simulink model "ESE4481_hw2 - Copy"  (R2021a)
settings: Solver=VariableStepAuto  StartTime=0.0  StopTime=10.0  RelTol=1e-3
undefined symbols (not defined in the file or in its folder): g, J, m, omega_0, p_ned_0, Theta_0, V_b_0
libraries: vrlib x4
settings Model: Creator=tomwh  LastModifiedBy=tomwh
settings DataIOCC: ExternalInput=F_b,omega_bE,M_b

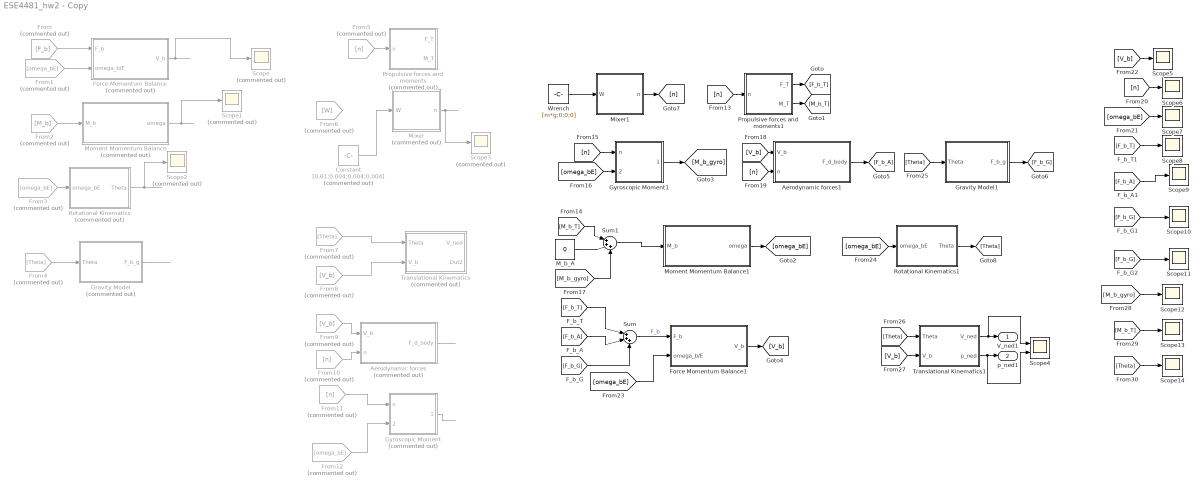
== system ESE4481_hw2 - Copy ==
  Aerodynamic forces : Subsystem  Commented=on
  Aerodynamic forces1 : Subsystem
  Constant : Constant  Commented=on  Value=[0.01;0.004;0.004;0.004]
  Force Momentum Balance : Subsystem  Commented=on
  Force Momentum Balance1 : Subsystem
  From : From  Commented=on  GotoTag=F_b
  From1 : From  Commented=on  GotoTag=omega_bE
  From10 : From  Commented=on  GotoTag=n
  From11 : From  Commented=on  GotoTag=n
  From12 : From  Commented=on  GotoTag=omega_bE
  From2 : From  Commented=on  GotoTag=M_b
  From3 : From  Commented=on  GotoTag=omega_bE
  From4 : From  Commented=on  GotoTag=Theta
  From5 : From  Commented=on  GotoTag=n
  From6 : From  Commented=on  GotoTag=W
  From7 : From  Commented=on  GotoTag=Theta
  From8 : From  Commented=on  GotoTag=V_b
  From9 : From  Commented=on  GotoTag=V_b
  Gravity Model : Subsystem  Commented=on
  Gravity Model1 : Subsystem
  Gyroscopic Moment : Subsystem  Commented=on
  Gyroscopic Moment1 : Subsystem
  M_b_A : Constant  Value=0
  Mixer : Subsystem  Commented=on
  Mixer1 : Subsystem
  Moment Momentum Balance : Subsystem  Commented=on
  Moment Momentum Balance1 : Subsystem
  Propulsive forces and moments : Subsystem  Commented=on
  Propulsive forces and moments1 : Subsystem
  Rotational Kinematics : Subsystem  Commented=on
  Rotational Kinematics1 : Subsystem
  Scope{,1..3} (4 alike) : Scope  Commented=on
  Scope{5..14} (10 alike) : Scope
  Scope4 : Scope  NumInputPorts=2
  Sum : Sum  Inputs=|+++
  Sum1 : Sum  Inputs=|+++
  Translational Kinematics : Subsystem  Commented=on
  Translational Kinematics1 : Subsystem
  Wrench : Constant  Value=[m*g;0;0;0]
  V_ned1 : Outport
  p_ned1 : Outport  Port=2
  wires:
  Force Momentum Balance/1(V_b) -> Scope/1
  From2/1 -> Moment Momentum Balance/1(M_b)
  Moment Momentum Balance/1(omega) -> Scope1/1
  Rotational Kinematics/1(Theta) -> Scope2/1
  From1/1 -> Force Momentum Balance/2(omega_b/E)
  From/1 -> Force Momentum Balance/1(F_b)
  From3/1 -> Rotational Kinematics/1(omega_bE)
  From4/1 -> Gravity Model/1(Theta)
  Gravity Model/1(F_b_g) -> ?
  From5/1 -> Propulsive forces and moments/1(n)
  Mixer/1(n) -> Scope3/1
  Constant/1 -> Mixer/1(W)
  From7/1 -> Translational Kinematics/1(Theta)
  From8/1 -> Translational Kinematics/2(V_b)
  From9/1 -> Aerodynamic forces/1(V_b)
  From10/1 -> Aerodynamic forces/2(n)
  Aerodynamic forces/1(F_d_body) -> ?
  Wrench/1 -> Mixer1/1(W)
  Mixer1/1(n) -> [n]
  [n] -> Propulsive forces and moments1/1(n)
  Propulsive forces and moments1/1(F_T) -> [F_b_T]
  Propulsive forces and moments1/2(M_T) -> [M_b_T]
  [M_b_T] -> Sum1/1
  M_b_A/1 -> Sum1/2
  From11/1 -> Gyroscopic Moment/1(n)
  From12/1 -> Gyroscopic Moment/2(omega_bE)
  Gyroscopic Moment/1(M_gyro) -> ?
  [n] -> Gyroscopic Moment1/1(n)
  Moment Momentum Balance1/1(omega) -> [omega_bE]
  [omega_bE] -> Gyroscopic Moment1/2(omega_bE)
  Gyroscopic Moment1/1(M_gyro) -> [M_b_gyro]
  Sum1/1 -> Moment Momentum Balance1/1(M_b)
  [M_b_gyro] -> Sum1/3
  Force Momentum Balance1/1(V_b) -> [V_b]
  [V_b] -> Aerodynamic forces1/1(V_b)
  [n] -> Aerodynamic forces1/2(n)
  Aerodynamic forces1/1(F_d_body) -> [F_b_A]
  Gravity Model1/1(F_b_g) -> [F_b_G]
  [F_b_T] -> Sum/1
  [F_b_A] -> Sum/2
  [F_b_G] -> Sum/3
  Sum/1 -> Force Momentum Balance1/1(F_b)  "F_b"
  [omega_bE] -> Force Momentum Balance1/2(omega_b/E)
  [omega_bE] -> Rotational Kinematics1/1(omega_bE)
  Rotational Kinematics1/1(Theta) -> [Theta]
  [Theta] -> Gravity Model1/1(Theta)
  [Theta] -> Translational Kinematics1/1(Theta)
  [V_b] -> Translational Kinematics1/2(V_b)
  Translational Kinematics1/2(p_ned) -> Scope4/2, p_ned1/1
  Translational Kinematics1/1(V_ned) -> Scope4/1, V_ned1/1
  [V_b] -> Scope5/1
  [n] -> Scope6/1
  [omega_bE] -> Scope7/1
  [F_b_T] -> Scope8/1
  [Theta] -> Scope14/1
  [M_b_T] -> Scope13/1
  [M_b_gyro] -> Scope12/1
  [F_b_G] -> Scope11/1
  [F_b_G] -> Scope10/1
  [F_b_A] -> Scope9/1

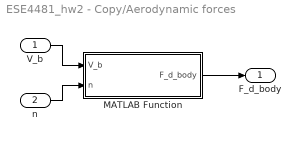
== system ESE4481_hw2 - Copy/Aerodynamic forces ==
  V_b : Inport
  n : Inport  Port=2
  MATLAB Function : MATLAB Function  TreatAsAtomicUnit=on
  F_d_body : Outport
  wires:
  MATLAB Function/1(F_d_body) -> F_d_body/1
  n/1 -> MATLAB Function/2(n)
  V_b/1 -> MATLAB Function/1(V_b)

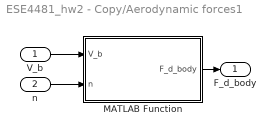
== system ESE4481_hw2 - Copy/Aerodynamic forces1 ==
  V_b : Inport
  n : Inport  Port=2
  MATLAB Function : MATLAB Function  TreatAsAtomicUnit=on
  F_d_body : Outport
  wires:
  MATLAB Function/1(F_d_body) -> F_d_body/1
  n/1 -> MATLAB Function/2(n)
  V_b/1 -> MATLAB Function/1(V_b)

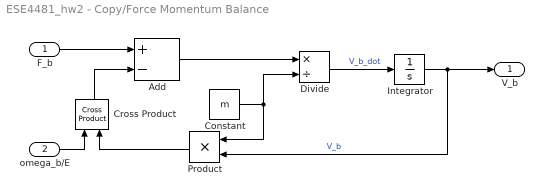
== system ESE4481_hw2 - Copy/Force Momentum Balance ==
  F_b : Inport
  omega_b/E : Inport  Port=2
  Add : Sum  Inputs=+-
  Constant : Constant  Value=m
  Cross Product : vrlib/Utilities/Cross Product
  Divide : Product  Inputs=*/
  Integrator : Integrator  InitialCondition=V_b_0
      settings: AttributesFormatString=%<InitialCondition>
  Product : Product
  V_b : Outport
  wires:
  omega_b/E/1 -> Cross Product/1
  F_b/1 -> Add/1
  Integrator/1 -> V_b/1, Product/2  "V_b"
  Constant/1 -> Divide/2, Product/1
  Divide/1 -> Integrator/1  "V_b_dot"
  Add/1 -> Divide/1
  Cross Product/1 -> Add/2
  Product/1 -> Cross Product/2

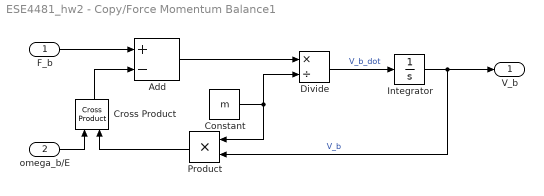
== system ESE4481_hw2 - Copy/Force Momentum Balance1 ==
  F_b : Inport
  omega_b/E : Inport  Port=2
  Add : Sum  Inputs=+-
  Constant : Constant  Value=m
  Cross Product : vrlib/Utilities/Cross Product
  Divide : Product  Inputs=*/
  Integrator : Integrator  InitialCondition=V_b_0
      settings: AttributesFormatString=%<InitialCondition>
  Product : Product
  V_b : Outport
  wires:
  omega_b/E/1 -> Cross Product/1
  F_b/1 -> Add/1
  Integrator/1 -> V_b/1, Product/2  "V_b"
  Constant/1 -> Divide/2, Product/1
  Divide/1 -> Integrator/1  "V_b_dot"
  Add/1 -> Divide/1
  Cross Product/1 -> Add/2
  Product/1 -> Cross Product/2

== system ESE4481_hw2 - Copy/Gravity Model ==
  Theta : Inport
  MATLAB Function : MATLAB Function  TreatAsAtomicUnit=on
  F_b_g : Outport
  wires:
  Theta/1 -> MATLAB Function/1(Theta)
  MATLAB Function/1(F_b_g) -> F_b_g/1

== system ESE4481_hw2 - Copy/Gravity Model1 ==
  Theta : Inport
  MATLAB Function : MATLAB Function  TreatAsAtomicUnit=on
  F_b_g : Outport
  wires:
  Theta/1 -> MATLAB Function/1(Theta)
  MATLAB Function/1(F_b_g) -> F_b_g/1

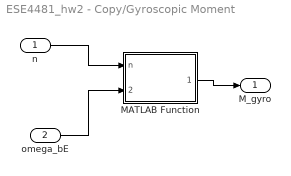
== system ESE4481_hw2 - Copy/Gyroscopic Moment ==
  n : Inport
  omega_bE : Inport  Port=2
  MATLAB Function : MATLAB Function  TreatAsAtomicUnit=on
  M_gyro : Outport
  wires:
  n/1 -> MATLAB Function/1(n)
  MATLAB Function/1(M_gyro) -> M_gyro/1
  omega_bE/1 -> MATLAB Function/2(omega_bE)

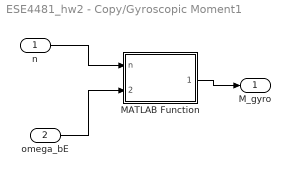
== system ESE4481_hw2 - Copy/Gyroscopic Moment1 ==
  n : Inport
  omega_bE : Inport  Port=2
  MATLAB Function : MATLAB Function  TreatAsAtomicUnit=on
  M_gyro : Outport
  wires:
  n/1 -> MATLAB Function/1(n)
  MATLAB Function/1(M_gyro) -> M_gyro/1
  omega_bE/1 -> MATLAB Function/2(omega_bE)

== system ESE4481_hw2 - Copy/Mixer ==
  W : Inport
  MATLAB Function : MATLAB Function  TreatAsAtomicUnit=on
  n : Outport
  wires:
  MATLAB Function/1(n) -> n/1
  W/1 -> MATLAB Function/1(W)

== system ESE4481_hw2 - Copy/Mixer1 ==
  W : Inport
  MATLAB Function : MATLAB Function  TreatAsAtomicUnit=on
  n : Outport
  wires:
  MATLAB Function/1(n) -> n/1
  W/1 -> MATLAB Function/1(W)

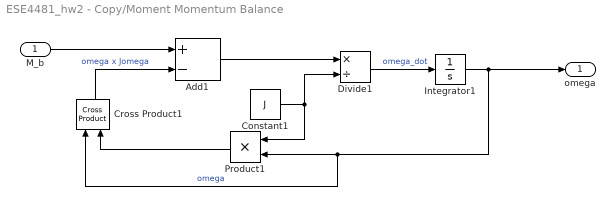
== system ESE4481_hw2 - Copy/Moment Momentum Balance ==
  M_b : Inport
  Add1 : Sum  Inputs=+-
  Constant1 : Constant  Value=J
  Cross Product1 : vrlib/Utilities/Cross Product
  Divide1 : Product  Inputs=*/
  Integrator1 : Integrator  InitialCondition=omega_0
      settings: AttributesFormatString=%<InitialCondition>
  Product1 : Product
  omega : Outport
  wires:
  Constant1/1 -> Divide1/2, Product1/1
  Cross Product1/1 -> Add1/2  "omega x Jomega"
  Integrator1/1 -> omega/1, Cross Product1/1, Product1/2  "omega"
  Product1/1 -> Cross Product1/2
  Add1/1 -> Divide1/1
  Divide1/1 -> Integrator1/1  "omega_dot"
  M_b/1 -> Add1/1

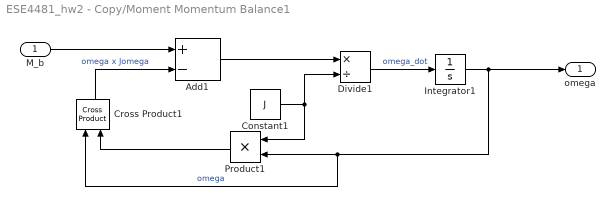
== system ESE4481_hw2 - Copy/Moment Momentum Balance1 ==
  M_b : Inport
  Add1 : Sum  Inputs=+-
  Constant1 : Constant  Value=J
  Cross Product1 : vrlib/Utilities/Cross Product
  Divide1 : Product  Inputs=*/
  Integrator1 : Integrator  InitialCondition=omega_0
      settings: AttributesFormatString=%<InitialCondition>
  Product1 : Product
  omega : Outport
  wires:
  Constant1/1 -> Divide1/2, Product1/1
  Cross Product1/1 -> Add1/2  "omega x Jomega"
  Integrator1/1 -> omega/1, Cross Product1/1, Product1/2  "omega"
  Product1/1 -> Cross Product1/2
  Add1/1 -> Divide1/1
  Divide1/1 -> Integrator1/1  "omega_dot"
  M_b/1 -> Add1/1

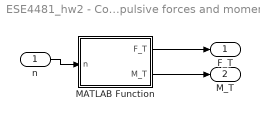
== system ESE4481_hw2 - Copy/Propulsive forces and moments ==
  n : Inport
  MATLAB Function : MATLAB Function  TreatAsAtomicUnit=on
  F_T : Outport
  M_T : Outport  Port=2
  wires:
  MATLAB Function/2(M_T) -> M_T/1
  n/1 -> MATLAB Function/1(n)
  MATLAB Function/1(F_T) -> F_T/1

== system ESE4481_hw2 - Copy/Propulsive forces and moments1 ==
  n : Inport
  MATLAB Function : MATLAB Function  TreatAsAtomicUnit=on
  F_T : Outport
  M_T : Outport  Port=2
  wires:
  MATLAB Function/2(M_T) -> M_T/1
  n/1 -> MATLAB Function/1(n)
  MATLAB Function/1(F_T) -> F_T/1

== system ESE4481_hw2 - Copy/Rotational Kinematics ==
  omega_bE : Inport
  Integrator : Integrator  InitialCondition=Theta_0
      settings: AttributesFormatString=%<InitialCondition>
  MATLAB Function : MATLAB Function  TreatAsAtomicUnit=on
  Theta : Outport
  wires:
  Integrator/1 -> MATLAB Function/1(Theta), Theta/1  "Theta"
  omega_bE/1 -> MATLAB Function/2(omega_bE)
  MATLAB Function/1(Theta_dot) -> Integrator/1

== system ESE4481_hw2 - Copy/Rotational Kinematics1 ==
  omega_bE : Inport
  Integrator : Integrator  InitialCondition=Theta_0
      settings: AttributesFormatString=%<InitialCondition>
  MATLAB Function : MATLAB Function  TreatAsAtomicUnit=on
  Theta : Outport
  wires:
  Integrator/1 -> MATLAB Function/1(Theta), Theta/1  "Theta"
  omega_bE/1 -> MATLAB Function/2(omega_bE)
  MATLAB Function/1(Theta_dot) -> Integrator/1

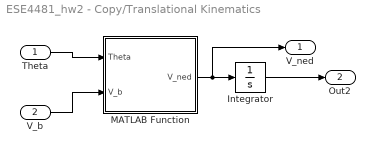
== system ESE4481_hw2 - Copy/Translational Kinematics ==
  Theta : Inport
  V_b : Inport  Port=2
  Integrator : Integrator  InitialCondition=p_ned_0
      settings: AttributesFormatString=%<InitialCondition>
  MATLAB Function : MATLAB Function  TreatAsAtomicUnit=on
  V_ned : Outport
  Out2 : Outport  Port=2
  wires:
  MATLAB Function/1(V_ned) -> V_ned/1, Integrator/1
  V_b/1 -> MATLAB Function/2(V_b)
  Integrator/1 -> Out2/1
  Theta/1 -> MATLAB Function/1(Theta)

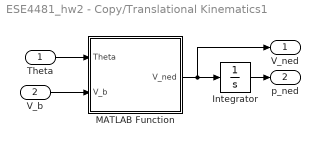
== system ESE4481_hw2 - Copy/Translational Kinematics1 ==
  Theta : Inport
  V_b : Inport  Port=2
  Integrator : Integrator  InitialCondition=p_ned_0
      settings: AttributesFormatString=%<InitialCondition>
  MATLAB Function : MATLAB Function  TreatAsAtomicUnit=on
  V_ned : Outport
  p_ned : Outport  Port=2
  wires:
  MATLAB Function/1(V_ned) -> V_ned/1, Integrator/1
  V_b/1 -> MATLAB Function/2(V_b)
  Integrator/1 -> p_ned/1
  Theta/1 -> MATLAB Function/1(Theta)

== matlab function ESE4481_hw2 - Copy/Rotational Kinematics1/MATLAB Function ==
  data: Theta input; Theta_dot output; omega_bE input
function Theta_dot = fcn(Theta,omega_bE)
    phi = Theta(1);
    theta = Theta(1);
    H_inv = [1 sin(phi)*tan(theta) cos(phi)*tan(theta);
             0 cos(phi) -sin(phi);
             0 sin(phi)*sec(theta) cos(phi)*sec(theta)];
Theta_dot = H_inv*omega_bE;

== matlab function ESE4481_hw2 - Copy/Translational Kinematics1/MATLAB Function ==
  data: Theta input; V_ned output; V_b input
function V_ned = fcn(Theta,V_b)
phi = Theta(1);
theta = Theta(2);
psi = Theta(3);
R = [cos(psi)*cos(theta) cos(theta)*sin(psi) -sin(theta);
     cos(psi)*sin(phi)*sin(theta)-cos(phi)*sin(psi) cos(phi)*cos(psi)+sin(phi)*sin(psi)*sin(theta) cos(theta)*sin(phi)
     sin(phi)*sin(psi)+cos(phi)*cos(psi)*sin(theta) cos(phi)*sin(psi)*sin(theta)-cos(psi)*sin(phi) cos(phi)*cos(theta)];
V_ned = R\V_b;

== matlab function ESE4481_hw2 - Copy/Rotational Kinematics/MATLAB Function ==
  data: Theta input; Theta_dot output; omega_bE input
function Theta_dot = fcn(Theta,omega_bE)
    phi = Theta(1);
    theta = Theta(1);
    H_inv = [1 sin(phi)*tan(theta) cos(phi)*tan(theta);
             0 cos(phi) -sin(phi);
             0 sin(phi)*sec(theta) cos(phi)*sec(theta)];
Theta_dot = H_inv*omega_bE;

== matlab function ESE4481_hw2 - Copy/Propulsive forces and moments/MATLAB Function ==
  data: n input; F_T output; M_T output
function [F_T,M_T]= fcn(n)
a = 2.3196*10^(-6);
b = 1.1047*10^(-7);
c = b;
d = 1.0566*10^(-8);
F_T = [0;0; -a*(n(1)^2 + n(2)^2 + n(3)^2 + n(4)^2)];
M_T = [b*(n(1)^2 - n(2)^2 - n(3)^2 + n(4)^2);c*(n(1)^2 + n(2)^2 - n(3)^2 - n(4)^2); d*(-n(1)^2 + n(2)^2 - n(3)^2 + n(4)^2)];

== matlab function ESE4481_hw2 - Copy/Mixer/MATLAB Function ==
  data: W input; n output
function n = getMotorSpeeds(W)
a = 2.3196*10^(-6);
b = 1.1047*10^(-7);
c = b;
d = 1.0566*10^(-8);
M = [a a a a;
    b -b -b b;
    c c -c -c;
    -d d -d d];
nu = abs(M\W);
n = sqrt(nu);

== matlab function ESE4481_hw2 - Copy/Translational Kinematics/MATLAB Function ==
  data: Theta input; V_ned output; V_b input
function V_ned = fcn(Theta,V_b)
phi = Theta(1);
theta = Theta(2);
psi = Theta(3);
R = [cos(psi)*cos(theta) cos(theta)*sin(psi) -sin(theta);
     cos(psi)*sin(phi)*sin(theta)-cos(phi)*sin(psi) cos(phi)*cos(psi)+sin(phi)*sin(psi)*sin(theta) cos(theta)*sin(phi)
     sin(phi)*sin(psi)+cos(phi)*cos(psi)*sin(theta) cos(phi)*sin(psi)*sin(theta)-cos(psi)*sin(phi) cos(phi)*cos(theta)];
V_ned = R*V_b;

== matlab function ESE4481_hw2 - Copy/Aerodynamic forces/MATLAB Function ==
  data: V_b input; F_d_body output; n input
function F_d_body = fcn(V_b,n)
rho = 1.293;
D = 0.066;
C_t = @(n) 4.375*10^(-5)*n + 0.0704;
K_c = 0.22;
K = [K_c 0 0;
     0 K_c 0;
     0 0 0];
F_d_body = -rho*C_t(abs(n(1)))*D^4*(n(1)^2 + n(2)^2 + n(3)^2 + n(4)^2)*K*V_b;

== matlab function ESE4481_hw2 - Copy/Gyroscopic Moment/MATLAB Function ==
  data: n input; M_gyro output; omega_bE input
function M_gyro = fcn(n,omega_bE)
    J = 1.2657*10^(-5);
    H = [0;0; J*2*pi*(n(1)-n(2)+n(3)-n(4))];
M_gyro = cross(omega_bE,H);

== matlab function ESE4481_hw2 - Copy/Mixer1/MATLAB Function ==
  data: W input; n output
function n = getMotorSpeeds(W)
a = 2.3196*10^(-6);
b = 1.1047*10^(-7);
c = b;
d = 1.0566*10^(-8);
M = [a a a a;
    b -b -b b;
    c c -c -c;
    -d d -d d];
nu = abs(M\W);
n = sqrt(nu);

== matlab function ESE4481_hw2 - Copy/Propulsive forces and moments1/MATLAB Function ==
  data: n input; F_T output; M_T output
    function [F_T,M_T]= fcn(n)
a = 2.3196*10^(-6);
b = 1.1047*10^(-7);
c = b;
d = 1.0566*10^(-8);
F_T = [0;0; -a*(n(1)^2 + n(2)^2 + n(3)^2 + n(4)^2)];
M_T = [b*(n(1)^2 - n(2)^2 - n(3)^2 + n(4)^2);c*(n(1)^2 + n(2)^2 - n(3)^2 - n(4)^2); d*(-n(1)^2 + n(2)^2 - n(3)^2 + n(4)^2)];

== matlab function ESE4481_hw2 - Copy/Aerodynamic forces1/MATLAB Function ==
  data: V_b input; F_d_body output; n input
function F_d_body = fcn(V_b,n)
rho = 1.293;
D = 0.066;
C_t = @(n) 4.375*10^(-5)*n + 0.0704;
K_c = 0.22;
K = [K_c 0 0;
     0 K_c 0;
     0 0 0];
F_d_body = -rho*C_t(abs(n(1)))*D^4*(n(1)^2 + n(2)^2 + n(3)^2 + n(4)^2)*K*V_b;

== matlab function ESE4481_hw2 - Copy/Gyroscopic Moment1/MATLAB Function ==
  data: n input; M_gyro output; omega_bE input
function M_gyro = fcn(n,omega_bE)
    J = 1.2657*10^(-5);
    H = [0;0; J*2*pi*(n(1)-n(2)+n(3)-n(4))];
M_gyro = cross(omega_bE,H);

== matlab function ESE4481_hw2 - Copy/Gravity Model/MATLAB Function ==
  data: Theta input; F_b_g output
function F_b_g = fcn(Theta)
phi = Theta(1);
theta = Theta(1);
R_b_E = [cos(theta) 0 -sin(theta);
         sin(phi)*sin(theta) cos(phi) cos(theta)*sin(phi);
         cos(phi)*sin(theta) -sin(phi) cos(theta)*cos(phi)];
m = 0.066;
g = 9.81;
F_b_g = R_b_E*[0; 0; m*g];

== matlab function ESE4481_hw2 - Copy/Gravity Model1/MATLAB Function ==
  data: Theta input; F_b_g output
function F_b_g = fcn(Theta)
phi = Theta(1);
theta = Theta(1);
R_b_E = [cos(theta) 0 -sin(theta);
         sin(phi)*sin(theta) cos(phi) cos(theta)*sin(phi);
         cos(phi)*sin(theta) -sin(phi) cos(theta)*cos(phi)];
m = 0.066;
g = 9.81;   
F_b_g = R_b_E*[0; 0; m*g];
